simulink model "Model"  (R2023b)
settings: Solver=VariableStepAuto  StartTime=0.0  StopTime=10.0  RelTol=1e-3
undefined symbols (not defined in the file): Brake, Gear, HandBrake, ManualGearShift, Reverse, Steer, Throttle
libraries: robotlib x8, sldrtlib x1, mpcadaslib x1
settings Model: Creator=EcoCAR  LastModifiedBy=EcoCAR

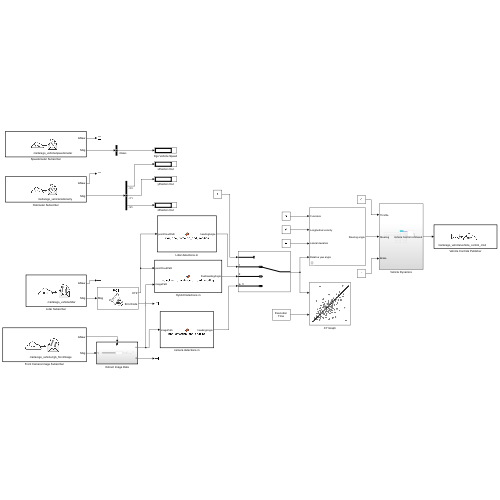
[thumbnail: Simulink's stored preview of the top-level diagram]
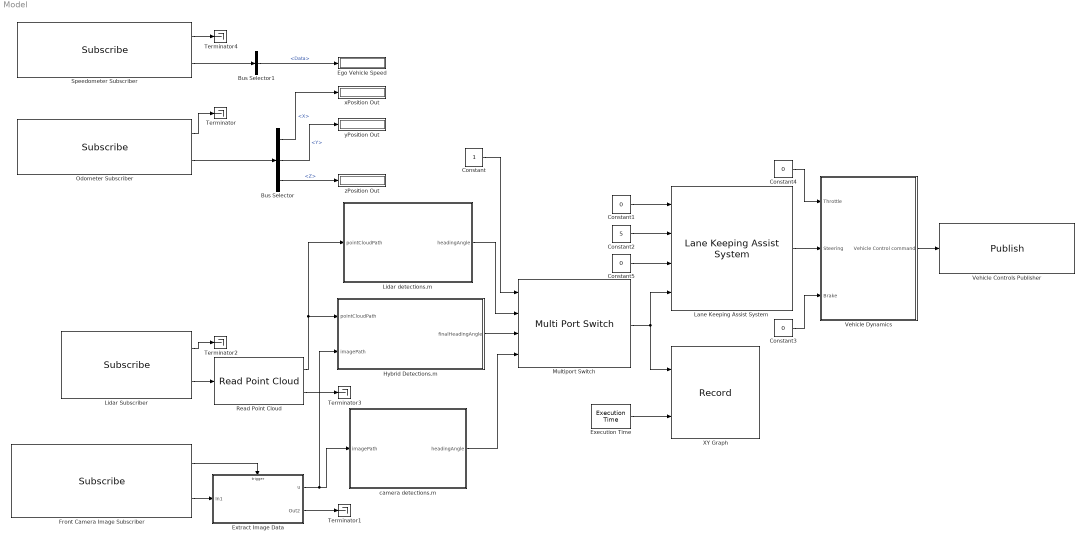
== system Model ==
  Bus Selector : BusSelector  DialogController=Simulink.DDGSource_BusSelector  OutputSignals=Pose.Pose.Position.X,Pose.Pose.Position.Y,Pose.Pose.Position.Z
  Bus Selector1 : BusSelector  OutputSignals=Data
  Constant : Constant
  Constant{1,3..5} (4 alike) : Constant  Value=0
  Constant2 : Constant  Value=5
  Ego Vehicle Speed : Display
  Execution Time : sldrtlib/Target Profiling/Execution Time  ShowTaskTimes=off
  Extract Image Data : Subsystem
  Front Camera Image Subscriber : robotlib/Subscribe  topicSource=Select from ROS network  topic=/carla/ego_vehicle/rgb_front/image  messageType=sensor_msgs/Image  SampleTime=-1  legacyBusStruct=off  messageQueueLength=1
  Hybrid Detections.m : MATLAB Function  TreatAsAtomicUnit=on
  Lane Keeping Assist System : mpcadaslib/Lane Keeping Assist System  ModelType=Use vehicle parameters  VehicleMass=1575  VehicleYawInertia=2875  LengthToFront=1.2  LengthToRear=1.6  FrontTireStiffness=19000  RearTireStiffness=33000  EgoModelMatrixA=[-4.4021 ,-12.4603;1.3913,-5.1868]  EgoModelMatrixB=[24.1270;15.8609]  EgoModelMatrixC=[1,0;0,1]  InitialLongVel=15  TransportLag=0  MinSteering=-0.26  umin_ext=off  MaxSteering=0.26  umax_ext=off  Ts=0.1  PredictionHorizon=10  ControllerBehavior=0.5  suboptimal=off  maxiter=10  datatypeopt=double  optmode=off  trackmode=off
      settings: LibrarySourceBlock=mpclib/Automated Driving/Lane Keeping Assist System
  Lidar Subscriber : robotlib/Subscribe  topicSource=Select from ROS network  topic=/carla/ego_vehicle/lidar  messageType=sensor_msgs/PointCloud2  SampleTime=-1  legacyBusStruct=off  messageQueueLength=1
  Lidar detections.m : MATLAB Function  TreatAsAtomicUnit=on
  Multiport Switch : MultiPortSwitch  SaturateOnIntegerOverflow=off  InputSameDT=off
  Odometer Subscriber : robotlib/Subscribe  topicSource=Select from ROS network  topic=/carla/ego_vehicle/odometry  messageType=nav_msgs/Odometry  SampleTime=-1  legacyBusStruct=off  messageQueueLength=1
  Read Point Cloud : robotlib/Read Point Cloud  MaximumPointCloudSize=[ 480, 640 ]  PreserveStructure=off  ShowRGBOutput=off  ShowIntensityOutput=off  ShowErrorCodeOutput=on  VariableSizeOutputs=off
  Speedometer Subscriber : robotlib/Subscribe  topicSource=Select from ROS network  topic=/carla/ego_vehicle/speedometer  messageType=std_msgs/Float32  SampleTime=-1  legacyBusStruct=off  messageQueueLength=1
  Terminator{,1..4} (5 alike) : Terminator
  Vehicle Controls Publisher : robotlib/Publish  topicSource=Specify your own  topic=/carla/ego_vehicle/vehicle_control_cmd  messageType=carla_msgs/CarlaEgoVehicleControl  legacyBusStruct=off  messageQueueLength=1
  Vehicle Dynamics : Subsystem
  XY Graph : Record  FileSettingsInternal="{\"entries\":[{\"content\":{\"excelSettings\":{\"content\":{},\"type\":\"Streamout.ExcelSettings\"}},\"type\":\"Streamout.FileSettingStorage\",\"uuid\":\"\"}],\"packageUris\":[\"http:\\/\\/schema.mathworks.com\\/mf0\\/streamout_blocks\\/R2020a\"],\"version\":\"1.0\"}"  Layout=[1 1]  SignalsInternal="{\"entries\":[{\"content\":{\"signals\":[{\"content\":{\"blockPath\":[],\"dimensions\":[1],\"domain\":\"\",\"lineColor\":\"#a2142f\",\"plots\":[1],\"port\":1,\"signalID\":60,\"signalName\":\"XY Graph:1\"},\"type\":\"RecordBlkView.Signal\",\"uuid\":\"\"},{\"content\":{\"blockPath\":[],\"dimensions\":[1],\"domain\":\"\",\"lineColor\":\"#139fff\",\"plots\":[1],\"port\":2,\"signalID\":63,\"signalName\":\"XY Graph:2\"},\"type\":\"RecordBlkView.Signal\",\"uuid\":\"\"}]},\"type\":\"RecordBlkView.InputSignals\",\"uuid\":\"\"}],\"packageUris\":[\"http:\\/\\/schema.mathworks.com\\/mf0\\/streamout_blocks\\/R2020a\"],\"version\":\"1.0\"}"  VisualizationBindings="{\"xyplotplugin\":{\"info\":[{\"series\":[{\"bindingParametersList\":[{\"parameter\":\"X-Axis\",\"signalID\":60,\"signalName\":\"XY Graph:1\"},{\"parameter\":\"Y-Axis\",\"signalID\":63,\"signalName\":\"XY Graph:2\"}],\"seriesID\":19023}],\"subplotID\":1}]}}"  CompatibilityTag=XY
  camera detections.m : MATLAB Function  TreatAsAtomicUnit=on
  xPosition Out : Display
  yPosition Out : Display
  zPosition Out : Display
  wires:
  Odometer Subscriber/2 -> Bus Selector/1
  Speedometer Subscriber/1 -> Terminator4/1
  Odometer Subscriber/1 -> Terminator/1
  Speedometer Subscriber/2 -> Bus Selector1/1
  Constant5/1 -> Lane Keeping Assist System/3
  Lidar Subscriber/1 -> Terminator2/1
  Front Camera Image Subscriber/2 -> Extract Image Data/1(In1)
  Extract Image Data/1(u) -> Hybrid Detections.m/2(imagePath), camera detections.m/1(imagePath)
  Front Camera Image Subscriber/1 -> Extract Image Data/Trigger
  Constant1/1 -> Lane Keeping Assist System/1
  Lidar Subscriber/2 -> Read Point Cloud/1
  Bus Selector1/1 -> Ego Vehicle Speed/1  "<Data>"
  Bus Selector/1 -> xPosition Out/1  "<X>"
  Bus Selector/2 -> yPosition Out/1  "<Y>"
  camera detections.m/1(headingAngle) -> Multiport Switch/4
  Read Point Cloud/2 -> Terminator3/1
  Bus Selector/3 -> zPosition Out/1  "<Z>"
  Read Point Cloud/1 -> Lidar detections.m/1(pointCloudPath), Hybrid Detections.m/1(pointCloudPath)
  Extract Image Data/2(Out2) -> Terminator1/1
  Constant/1 -> Multiport Switch/1
  Lidar detections.m/1(headingAngle) -> Multiport Switch/2
  Hybrid Detections.m/1(finalHeadingAngle) -> Multiport Switch/3
  Constant2/1 -> Lane Keeping Assist System/2
  Multiport Switch/1 -> XY Graph/1, Lane Keeping Assist System/4
  Execution Time/1 -> XY Graph/2
  Constant4/1 -> Vehicle Dynamics/1(Throttle)
  Lane Keeping Assist System/1 -> Vehicle Dynamics/2(Steering)
  Constant3/1 -> Vehicle Dynamics/3(Brake)
  Vehicle Dynamics/1(Vehicle Control command) -> Vehicle Controls Publisher/1

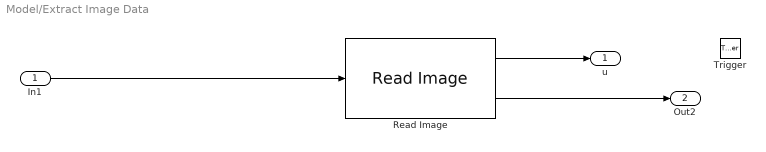
== system Model/Extract Image Data ==
  In1 : Inport
  Trigger : TriggerPort  VariantControl=(inherit)  PortDimensions=1
  Read Image : robotlib/Read Image  MaximumImageSize=[600, 800]  ImageEncoding=bgra8  ShowAlphaOutput=off  ShowErrorCodeOutput=on  VariableSizeOutputs=off
  u : Outport
  Out2 : Outport  Port=2
  wires:
  In1/1 -> Read Image/1
  Read Image/2 -> Out2/1
  Read Image/1 -> u/1

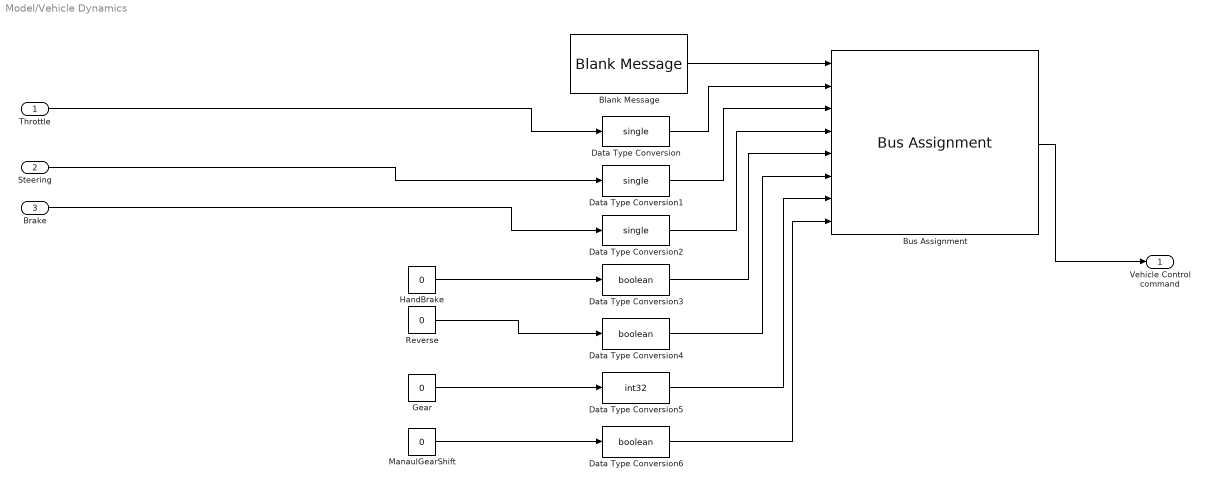
== system Model/Vehicle Dynamics ==
  Throttle : Inport
  Steering : Inport  Port=2
  Brake : Inport  Port=3
  Blank Message : robotlib/Blank Message  messageClass=Message  entityType=carla_msgs/CarlaEgoVehicleControl  messageType=carla_msgs/CarlaEgoVehicleControl  SampleTime=inf  legacyBusStruct=off
  Bus Assignment : BusAssignment  AssignedSignals=Throttle,Steer,Brake,HandBrake,Reverse,Gear,ManualGearShift
  Data Type Conversion : DataTypeConversion  OutDataTypeStr=single  SaturateOnIntegerOverflow=off  RndMeth=Floor
  Data Type Conversion1 : DataTypeConversion  OutDataTypeStr=single  SaturateOnIntegerOverflow=off  RndMeth=Floor
  Data Type Conversion2 : DataTypeConversion  OutDataTypeStr=single  SaturateOnIntegerOverflow=off  RndMeth=Floor
  Data Type Conversion3 : DataTypeConversion  OutDataTypeStr=boolean  SaturateOnIntegerOverflow=off  RndMeth=Floor
  Data Type Conversion4 : DataTypeConversion  OutDataTypeStr=boolean  SaturateOnIntegerOverflow=off  RndMeth=Floor
  Data Type Conversion5 : DataTypeConversion  OutDataTypeStr=int32  SaturateOnIntegerOverflow=off  RndMeth=Floor
  Data Type Conversion6 : DataTypeConversion  OutDataTypeStr=boolean  SaturateOnIntegerOverflow=off  RndMeth=Floor
  Gear : Constant  Value=0
  HandBrake : Constant  Value=0
  ManaulGearShift : Constant  Value=0
  Reverse : Constant  Value=0
  Vehicle Control command : Outport
  wires:
  ManaulGearShift/1 -> Data Type Conversion6/1
  Data Type Conversion2/1 -> Bus Assignment/4
  Data Type Conversion5/1 -> Bus Assignment/7
  Data Type Conversion/1 -> Bus Assignment/2
  Reverse/1 -> Data Type Conversion4/1
  Data Type Conversion4/1 -> Bus Assignment/6
  Brake/1 -> Data Type Conversion2/1
  Data Type Conversion1/1 -> Bus Assignment/3
  Steering/1 -> Data Type Conversion1/1
  Throttle/1 -> Data Type Conversion/1
  Data Type Conversion3/1 -> Bus Assignment/5
  Data Type Conversion6/1 -> Bus Assignment/8
  HandBrake/1 -> Data Type Conversion3/1
  Blank Message/1 -> Bus Assignment/1
  Bus Assignment/1 -> Vehicle Control command/1
  Gear/1 -> Data Type Conversion5/1

== matlab function Model/camera detections.m ==
  data: imagePath input; headingAngle output
function headingAngle = lane_detection_and_heading(imagePath)
    % Read an Frame
    frame = imread(imagePath); % Load the image

    % Process the image to detect lane lines
    lines = detectLaneLines(frame);

    % Calculate the trajectory
    trajectory = calculateTrajectory(lines, size(frame, 1));

    % Calculate the heading angle
    headingAngle = calculateHeadingAngle(trajectory);

    % Visualize the result
    visualizeResult(frame, lines, trajectory);
end

function lines = detectLaneLines(frame)
    % Convert to Grayscale
    gray = rgb2gray(frame);

    % Apply Gaussian Blur
    blurred = imgaussfilt(gray, 2);

    % Edge Detection
    edges = edge(blurred, 'Canny');

    % Define Region of Interest (ROI)
    roi = [0, size(edges,1); size(edges,2), size(edges,1); size(edges,2)/2, size(edges,1)/2];
    mask = poly2mask(roi(:,1), roi(:,2), size(edges,1), size(edges,2));
    maskedEdges = edges & mask;

    % Hough Transform for Line Detection
    [H, theta, rho] = hough(maskedEdges);
    peaks = houghpeaks(H, 5, 'threshold', ceil(0.3*max(H(:))));
    lines = houghlines(maskedEdges, theta, rho, peaks, 'FillGap', 20, 'MinLength', 30);
end

function trajectory = calculateTrajectory(lines, imageHeight)
    % Initialize an array to hold the center points of the lane
    laneCenters = [];

    % Iterate over a range of y-values (vertical positions in the image)
    for y = imageHeight:-10:0
        xPositions = [];

        % For each line, calculate the x-position at the current y-value
        for k = 1:length(lines)
            % Get the start and end points of the line
            p1 = lines(k).point1;
            p2 = lines(k).point2;

            % Check if the line crosses the current y-value
            if (p1(2) - y) * (p2(2) - y) < 0
                % Interpolate the x-position at the current y-value
                x = interp1([p1(2), p2(2)], [p1(1), p2(1)], y);
                xPositions(end + 1) = x;
            end
        end

        % Calculate the average x-position (center of the lane) at this y-value
        if ~isempty(xPositions)
            laneCenter = mean(xPositions);
            laneCenters = [laneCenters; [laneCenter, y]];
        end
    end

    % Return the calculated trajectory
    trajectory = laneCenters;
end

function headingAngle = calculateHeadingAngle(trajectory)
    if size(trajectory, 1) < 2
        headingAngle = NaN; % Cannot calculate angle
        return;
    end
    deltaY = trajectory(end, 2) - trajectory(1, 2);
    deltaX = trajectory(end, 1) - trajectory(1, 1);
    headingAngle = atan2(deltaY, deltaX); % Angle in radians
end


function visualizeResult(frame, lines, trajectory)
    figure, imshow(frame), hold on;
    for k = 1:length(lines)
        xy = [lines(k).point1; lines(k).point2];
        plot(xy(:,1), xy(:,2), 'LineWidth', 2, 'Color', 'green');
    end
    plot(trajectory(:,1), trajectory(:,2), 'LineWidth', 2, 'Color', 'blue');
    hold off;
end

== matlab function Model/Hybrid Detections.m ==
  data: pointCloudPath input; finalHeadingAngle output; imagePath input
function finalHeadingAngle = combined_lane_detection_and_heading(pointCloudPath, imagePath)
    % Process LIDAR data
    [lidarHeadingAngle, lidarTrajectory] = lidar_lane_detection_and_heading(pointCloudPath);

    % Process Camera data
    [cameraHeadingAngle, cameraTrajectory] = lane_detection_and_heading(imagePath);

    % Merge Trajectories
    mergedTrajectory = mergeTrajectories(lidarTrajectory, cameraTrajectory);

    % Calculate Final Steering Angle
    finalHeadingAngle = calculateFinalHeadingAngle(mergedTrajectory);
end

function headingAngle = lidar_lane_detection_and_heading(pointCloudPath)

    % Load LiDAR Point Cloud
    ptCloud = pcread(pointCloudPath); % Load the point cloud

    % Validate Point Cloud
    if isempty(ptCloud)
        error('Point cloud data is empty or invalid.');
    end

    % Enhanced Data Preprocessing
    preprocessedData = preprocessPointCloud(ptCloud); % Call from LidarDetections.m

    % Process the point cloud to detect lane lines
    laneLines = detectLaneLinesFromPointCloud(preprocessedData); % Call from LidarDetections.m

    % Error handling if no lanes are detected
    if isempty(laneLines)
        headingAngle = NaN;
        warning('No lane lines detected.');
        return;
    end

    % Calculate the trajectory with noise reduction
    trajectory = calculateSmoothTrajectory(laneLines, size(ptCloud.Location, 1)); % Call from LidarDetections.m

    % Calculate the heading angle with additional error handling
    headingAngle = calculateHeadingAngle(trajectory); % Call from LidarDetections.m

    % Visualize the result with enhanced visualization
    visualizeLidarResult(ptCloud, laneLines, trajectory); % Call from LidarDetections.m
end


function [headingAngle, trajectory] = lane_detection_and_heading(imagePath)
    % Load the image
    frame = imread(imagePath); % Load the image

    % Process the image to detect lane lines
    lines = detectLaneLines(frame); % Call from CameraDetections.m

    % Calculate the trajectory
    trajectory = calculateTrajectory(lines, size(frame, 1)); % Call from CameraDetections.m

    % Calculate the heading angle
    headingAngle = calculateHeadingAngle(trajectory); % Call from CameraDetections.m

    % Visualize the result
    visualizeResult(frame, lines, trajectory); % Call from CameraDetections.m
end

function mergedTrajectory = mergeTrajectories(lidarTrajectory, cameraTrajectory)
    % lidarConfidence and cameraConfidence are values between 0 and 1 indicating the confidence of each sensors data can be tuned to balance detections
    lidarConfidence = 0.8;
    cameraConfidence = 0.2;

    % Normalize confidences
    totalConfidence = lidarConfidence + cameraConfidence;
    normalizedLidarConfidence = lidarConfidence / totalConfidence;
    normalizedCameraConfidence = cameraConfidence / totalConfidence;

    % Ensure that both trajectories have the same length
    % This is a simple resampling. For better results, consider interpolation methods.
    minLength = min(size(lidarTrajectory, 1), size(cameraTrajectory, 1));
    lidarTrajectory = lidarTrajectory(1:minLength, :);
    cameraTrajectory = cameraTrajectory(1:minLength, :);

    % Compute the weighted average of the trajectories
    mergedTrajectory = normalizedLidarConfidence * lidarTrajectory + normalizedCameraConfidence * cameraTrajectory;
end


% Function to calculate the final heading angle from the merged trajectory
function finalHeadingAngle = calculateFinalHeadingAngle(trajectory)
    finalHeadingAngle = calculateHeadingAngle(trajectory); % Reuse existing function
end

== matlab function Model/Lidar detections.m ==
  data: pointCloudPath input; headingAngle output
function headingAngle = lidar_lane_detection_and_heading(pointCloudPath)
    % Load LiDAR Point Cloud
    ptCloud = pcread(pointCloudPath); % Load the point cloud

    % Validate Point Cloud
    if isempty(ptCloud)
        error('Point cloud data is empty or invalid.');
    end

    % Enhanced Data Preprocessing
    preprocessedData = preprocessPointCloud(ptCloud);

    % Process the point cloud to detect lane lines
    laneLines = detectLaneLinesFromPointCloud(preprocessedData);

    % Error handling if no lanes are detected
    if isempty(laneLines)
        headingAngle = NaN;
        warning('No lane lines detected.');
        return;
    end

    % Calculate the trajectory with noise reduction
    trajectory = calculateSmoothTrajectory(laneLines, size(ptCloud.Location, 1));

    % Calculate the heading angle with additional error handling
    headingAngle = calculateHeadingAngle(trajectory);

    % Visualize the result with enhanced visualization
    visualizeLidarResult(ptCloud, laneLines, trajectory);
end

function preprocessedData = preprocessPointCloud(ptCloud)
    % Noise Reduction using Statistical Outlier Removal
    ptCloud = pcdenoise(ptCloud);

    % Outlier Removal based on Distance
    distances = pdist2(ptCloud.Location, mean(ptCloud.Location, 1));
    threshold = mean(distances) + 2*std(distances);
    validPoints = distances <= threshold;

    % Return preprocessed data
    preprocessedData = select(ptCloud, validPoints);
end


function trajectory = calculateSmoothTrajectory(lines, imageHeight)
    % Initialize an array for the lane centers
    laneCenters = [];

    % Iterate over y-values
    for y = imageHeight:-10:0
        xPositions = [];
        
        % Calculate x-positions for each line
        for k = 1:length(lines)
            p1 = lines(k).point1;
            p2 = lines(k).point2;

            % Line intersection with current y-value
            if (p1(2) - y) * (p2(2) - y) < 0
                x = interp1([p1(2), p2(2)], [p1(1), p2(1)], y);
                xPositions(end + 1) = x;
            end
        end

        % Average x-position for lane center
        if ~isempty(xPositions)
            laneCenter = mean(xPositions);
            laneCenters = [laneCenters; [laneCenter, y]];
        end
    end

    % Apply a smoothing spline to reduce noise
    splineFit = fit(laneCenters(:,2), laneCenters(:,1), 'smoothingspline');
    smoothPoints = feval(splineFit, laneCenters(:,2));

    % Return the smooth trajectory
    trajectory = [smoothPoints, laneCenters(:,2)];
end


function headingAngle = calculateHeadingAngle(trajectory)
    if size(trajectory, 1) < 2
        headingAngle = NaN; % Cannot calculate angle
        return;
    end
    deltaY = trajectory(end, 2) - trajectory(1, 2);
    deltaX = trajectory(end, 1) - trajectory(1, 1);
    headingAngle = atan2(deltaY, deltaX); % Angle in radians
end

function visualizeLidarResult(ptCloud, laneLines, trajectory)
    % Create a figure for visualization
    figure;

    % Plot the original point cloud
    pcshow(ptCloud);
    hold on;

    % Plot each detected lane line
    for k = 1:length(laneLines)
        line = laneLines(k);
        p1 = line.point1;
        p2 = line.point2;
        plot3([p1(1), p2(1)], [p1(2), p2(2)], [p1(3), p2(3)], 'LineWidth', 2, 'Color', 'r');
    end

    % Plot the trajectory
    if ~isempty(trajectory)
        plot3(trajectory(:,1), trajectory(:,2), zeros(size(trajectory, 1), 1), 'LineWidth', 2, 'Color', 'g');
    end

    % Adjust plot properties
    xlabel('X');
    ylabel('Y');
    zlabel('Z');
    title('LiDAR Data with Detected Lane Lines and Trajectory');
    grid on;
    hold off;
end


function laneLines = detectLaneLinesFromPointCloud(ptCloud)
    % Project LiDAR data onto a 2D plane
    projectedData = projectLiDARto2D(ptCloud);

    % Filter the projected data to enhance potential lane lines
    filteredData = filterForLaneLines(projectedData);

    % Detect lane lines using a line detection algorithm
    laneLines = detectLines(filteredData);
end

function projectedData = projectLiDARto2D(ptCloud)
    % Extract x, y, and z coordinates
    x = ptCloud.Location(:,1);
    y = ptCloud.Location(:,2);
    z = ptCloud.Location(:,3);

    projectedData = [x, y];

end

function filteredData = filterForLaneLines(data)
    % Example of a simple threshold filter to focus on areas
    % where lane lines are more likely to be located.
    laneLineThreshold = 0.5; 
    
    % Apply a spatial filter or thresholding operation
    filteredData = data(data(:,2) < laneLineThreshold, :);
end


function lines = detectLines(data)
    binaryImage = false(1000, 1000);
    indices = sub2ind(size(binaryImage), data(:,1), data(:,2));
    binaryImage(indices) = true;

    % Apply Hough Transform to detect lines
    [H, theta, rho] = hough(binaryImage);
    peaks = houghpeaks(H, 5, 'threshold', ceil(0.3*max(H(:))));
    lines = houghlines(binaryImage, theta, rho, peaks, 'FillGap', 20, 'MinLength', 30);
end
